simulink model "planta_2024"  (R2024a)
settings: Solver=VariableStepAuto  StartTime=0.0  StopTime=300  RelTol=1e-3
values from neighbouring files (symbols this model uses):
  angulo_inicial = theta_exp(1) * pi / 180    [anterior.m]    (also in datos_planta.m; planta_procedimiento.m)
  B = 1.812642814729166e-04    (= 0.000181264281473)    [PI_calculo.m]    (also in anterior.m = 0.00181520669083; datos_planta.m; definir_incertidumbre.m = ureal('B', 1.81e-4, 'Percentage', 20); hallar_PID.m = 0.00181520669083)
  I = 0.0362    [PI_calculo.m]    (also in anterior.m = 0.0361594958333; datos_planta.m = 0.00361084226042; definir_incertidumbre.m = ureal('I', 0.0362 , 'Percentage', 15); hallar_PID.m = 0.0361594958333)
  k = (m*g*l/(2*I) + m_adicional * g * l / I)    (= 0.872324904512)    [anterior.m]    (also in datos_planta.m = m*g*l*cosd(punto_operacion); hallar_PID.m; planta_procedimiento.m)
  K_pwm_rad = 0.0382    [datos_planta.m]
  K_rad_grados = 180 / pi    (= 57.2957795131)    [anterior.m]    (also in datos_planta.m; planta_procedimiento.m)
  l = 0.145    [anterior.m]    (also in datos_planta.m; hallar_PID.m; planta_procedimiento.m)
settings Model: Creator=sergi  LastModifiedBy=sergi
settings ConfigComp: CovBoundaryAbsTol=1.0e-5

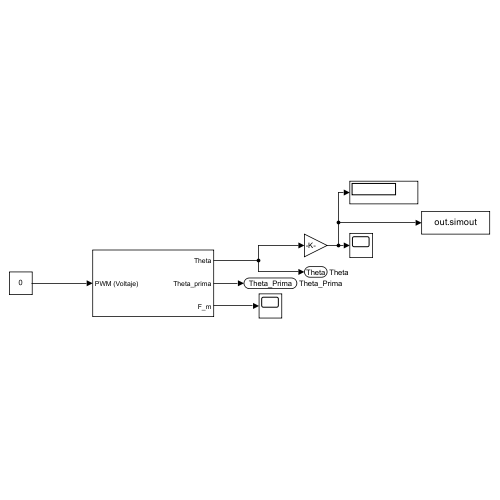
[thumbnail: Simulink's stored preview of the top-level diagram]
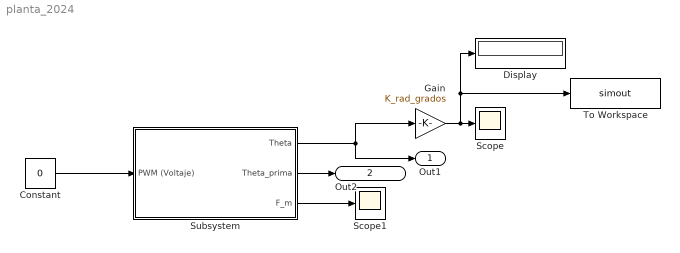
== system planta_2024 ==
  Constant : Constant  Value=0
  Display : Display
  Gain : Gain  Gain=K_rad_grados
  Scope : Scope
  Scope1 : Scope
  Subsystem : Subsystem
  To Workspace : ToWorkspace  VariableName=simout  SaveFormat=Timeseries  SampleTime=-1
  Out1 : Outport  SignalName=Theta
  Out2 : Outport  Port=2  SignalName=Theta_Prima
  wires:
  Constant/1 -> Subsystem/1(PWM (Voltaje))
  Subsystem/1(Theta) -> Out1/1, Gain/1
  Subsystem/2(Theta_prima) -> Out2/1
  Gain/1 -> To Workspace/1, Display/1, Scope/1
  Subsystem/3(F_m) -> Scope1/1

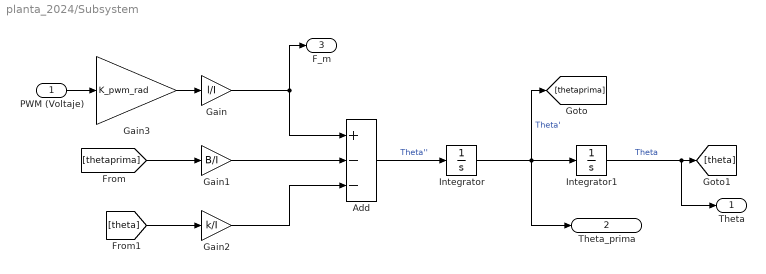
== system planta_2024/Subsystem ==
  PWM (Voltaje) : Inport
  Add : Sum  Inputs=+--
  Gain : Gain  Gain=l/I
  Gain1 : Gain  Gain=B/I
  Gain2 : Gain  Gain=k/I
  Gain3 : Gain  Gain=K_pwm_rad
  Integrator : Integrator
  Integrator1 : Integrator  InitialCondition=angulo_inicial
  Theta : Outport
  Theta_prima : Outport  Port=2
  F_m : Outport  Port=3
  wires:
  Gain2/1 -> Add/3
  [thetaprima] -> Gain1/1
  Add/1 -> Integrator/1  "Theta''"
  PWM (Voltaje)/1 -> Gain3/1
  Integrator/1 -> Theta_prima/1, [thetaprima], Integrator1/1  "Theta'"
  Integrator1/1 -> Theta/1, [theta]  "Theta"
  Gain3/1 -> Gain/1
  Gain/1 -> F_m/1, Add/1
  Gain1/1 -> Add/2
  [theta] -> Gain2/1
